simulink model "Sim1dot0"  (R2023b)
settings: Solver=VariableStepAuto  StartTime=0.0  StopTime=10.0  RelTol=1e-3
values from neighbouring files (symbols this model uses):
  dt = 0.02    [para_sim1dot0.mat]    (also in para_sim1dot1.mat; para_sim1dot2.mat; para_sim1dot3.mat; para_sim1dot4.mat)
  k_comp_1 = 1    [para_sim1dot0.mat]    (also in para_sim1dot1.mat; para_sim1dot2.mat; para_sim1dot3.mat; para_sim1dot4.mat)
  k_comp_2 = 1    [para_sim1dot0.mat]    (also in para_sim1dot1.mat; para_sim1dot2.mat; para_sim1dot3.mat; para_sim1dot4.mat)
  mass = 1    [para_sim1dot0.mat]    (also in para_sim1dot1.mat; para_sim1dot2.mat = 0.6; para_sim1dot3.mat = 0.8; para_sim1dot4.mat = 0.8)
  max_fin_angle_deg = 30    [para_sim1dot0.mat]    (also in para_sim1dot1.mat; para_sim1dot2.mat; para_sim1dot3.mat; para_sim1dot4.mat)
  v_min_controllable = 20    [para_sim1dot0.mat]    (also in para_sim1dot1.mat; para_sim1dot2.mat; para_sim1dot3.mat; para_sim1dot4.mat)
undefined symbols (not defined in the file or in its folder): DiscIntNeverNeededParam, state
libraries: robotcorelib x4, simulink x3, slpidlib x3, shared6dof x2, simulink_extras x2, aerolibutil x1, dspstat3 x1
settings Model: Creator=Zian Liu  LastModifiedBy=Zian Liu

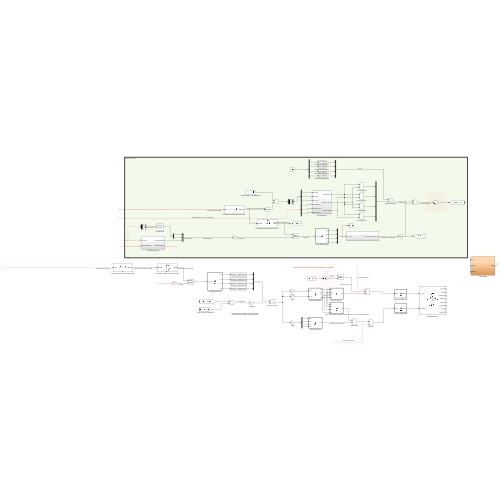
[thumbnail: Simulink's stored preview of the top-level diagram]
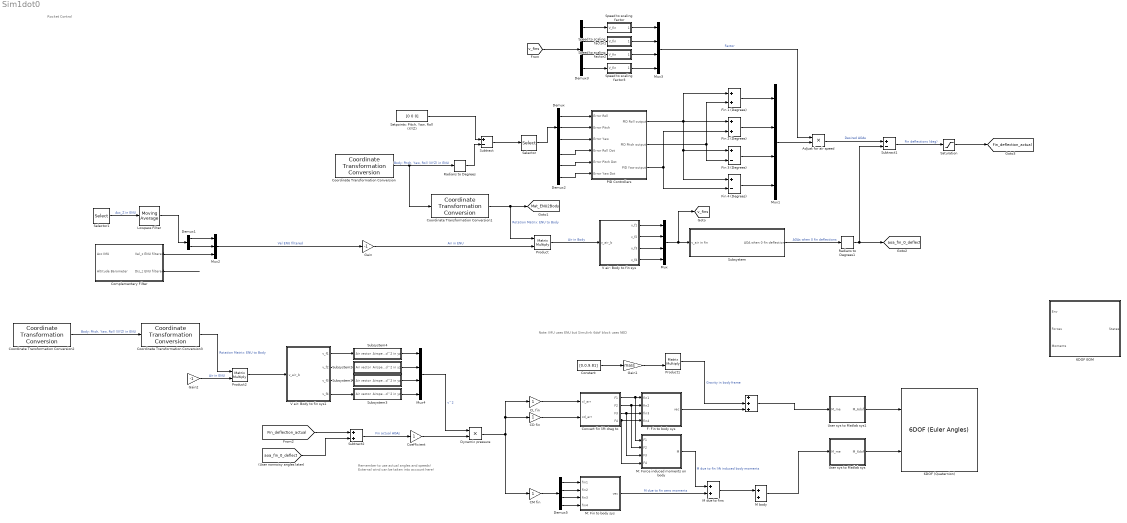
== system Sim1dot0 ==
  note: Note: IMU uses ENU but Simulink 6dof block uses NED
  note: Remember to use actual angles and speeds!
      | External wind can be taken into account here!
  note: Rocket Control
  " " : Sum  Inputs=+++
  6DOF (Quaternion) : shared6dof/6DOF (Euler Angles)  units=Metric (MKS)  mtype=Fixed  rep=Quaternion  xme_0=[0 0 0]  Vm_0=[0 0 0]  eul_0=[0 0 0]  pm_0=[0 0 0]  mass_0=1.0  mass_e=0.5  mass_f=2.0  inertia=eye(3)  inertia_e=eye(3)  inertia_f=2*eye(3)  k_quat=1.0  vre_flag=on  abi_flag=off  aMode=0  xme_statename=''  Vm_statename=''  eul_statename=''  quat_statename=''  pm_statename=''  mass_statename=''
      settings: LibrarySourceBlock=aerolib6dof2/6DOF (Quaternion)
  6DOF EOM : Subsystem  VariantControl=eom3DOF
  Adjust for air speed : Product
  CD fin : Gain
  CL fin : Gain
  CM fin : Gain
  Coefficient : Gain
  Complementary Filter : Subsystem
  Constant : Constant  Value=[0,0,9.81]
  "Convert fin lift drag to " : MATLAB Function  TreatAsAtomicUnit=on
  Coordinate Transformation Conversion : robotcorelib/Coordinate Transformation Conversion  InputRepresentation=Quaternion  InputEulerSequence=ZYX  ShowTrVecInputPort=on  OutputRepresentation=Euler Angles  OutputEulerSequence=XYZ  ShowTrVecOutputPort=on  SimulateUsing=Interpreted execution
      settings: LibrarySourceBlock=uavutilslib/Coordinate Transformation Conversion
  Coordinate Transformation Conversion1 : robotcorelib/Coordinate Transformation Conversion  InputRepresentation=Euler Angles  InputEulerSequence=XYZ  ShowTrVecInputPort=on  OutputRepresentation=Rotation Matrix  OutputEulerSequence=XYZ  ShowTrVecOutputPort=on  SimulateUsing=Interpreted execution
      settings: LibrarySourceBlock=uavutilslib/Coordinate Transformation Conversion
  Coordinate Transformation Conversion2 : robotcorelib/Coordinate Transformation Conversion  InputRepresentation=Quaternion  InputEulerSequence=ZYX  ShowTrVecInputPort=on  OutputRepresentation=Euler Angles  OutputEulerSequence=XYZ  ShowTrVecOutputPort=on  SimulateUsing=Interpreted execution
      settings: LibrarySourceBlock=uavutilslib/Coordinate Transformation Conversion
  Coordinate Transformation Conversion3 : robotcorelib/Coordinate Transformation Conversion  InputRepresentation=Euler Angles  InputEulerSequence=XYZ  ShowTrVecInputPort=on  OutputRepresentation=Rotation Matrix  OutputEulerSequence=XYZ  ShowTrVecOutputPort=on  SimulateUsing=Interpreted execution
      settings: LibrarySourceBlock=uavutilslib/Coordinate Transformation Conversion
  Demux : Demux  Outputs=3
  Demux1 : Demux  Outputs=2
  Demux2 : Demux  Outputs=3
  Demux3 : Demux
  Demux5 : Demux
  Dynamic pressure : Product
  F: Fin to body sys : MATLAB Function  TreatAsAtomicUnit=on
  Fin 1 (Degrees) : Sum
  Fin 2 (Degrees) : Sum
  Fin 3 (Degrees) : Sum  Inputs=+-
  Fin 4 (Degrees) : Sum  Inputs=+-
  Gain : Gain  Gain=-1
  Gain1 : Gain  Gain=mass
  Gain2 : Gain  Gain=-1
  Lowpass Filter : dspstat3/Moving Average  Method=Exponential weighting  ForgettingFactorPort=off  SpecifyWindowLength=on  WindowLength=4  OverlapLength=3  AllowArbitraryInputLength=off  ForgettingFactor=0.95  SimulateUsing=Code generation
  M body : Sum
  M due to fins : Sum
  M: Fin to body sys : MATLAB Function  TreatAsAtomicUnit=on
  M: Force induced moments on body : MATLAB Function  TreatAsAtomicUnit=on
  Mux{,1,3..4} (4 alike) : Mux
  Mux2 : Mux  Inputs=3
  PID Controllers : Subsystem
  Product : Product  Multiplication=Matrix(*)
  Product1 : Product  Multiplication=Matrix(*)
  Product2 : Product  Multiplication=Matrix(*)
  Radians to Degrees : simulink_extras/Transformations/Radians to Degrees
  Radians to Degrees1 : simulink_extras/Transformations/Radians to Degrees
  Saturation : Saturate  UpperLimit=max_fin_angle_deg  LowerLimit=-max_fin_angle_deg
  Selector : Selector  InputPortWidth=3  IndexOptions=Index vector (dialog)  Indices=[3 1 2]  OutputSizes=1
  Selector1 : Selector  InputPortWidth=3  IndexOptions=Index vector (dialog)  Indices=[1 2]  OutputSizes=1
  "Setpoints: Pitch, Yaw, Roll (XYZ)" : Constant  Value=[0 0 0]
  Speed to scaling factor : Subsystem
  Speed to scaling factor1 : Subsystem
  Speed to scaling factor2 : Subsystem
  Speed to scaling factor3 : Subsystem
  Subsystem : Subsystem
  Subsystem1 : Subsystem
  Subsystem2 : Subsystem
  Subsystem3 : Subsystem
  Subsystem4 : Subsystem
  Subtract : Sum  Inputs=+-
  Subtract1 : Sum  Inputs=+-
  Subtract2 : Sum
  User sys to Matlab sys : MATLAB Function  TreatAsAtomicUnit=on
  User sys to Matlab sys1 : MATLAB Function  TreatAsAtomicUnit=on
  V air: Body to fin sys : MATLAB Function  TreatAsAtomicUnit=on
  V air: Body to fin sys1 : MATLAB Function  TreatAsAtomicUnit=on
  tag scope: Fin_deflection_actual=global, Mat_ENU2Body=global, aoa_fin_0_deflect=global, v_fins=global
  wires:
  ? -> Coordinate Transformation Conversion/1  "Rocket attitude in quaternion"
  Coordinate Transformation Conversion/1 -> Coordinate Transformation Conversion1/1, Radians to Degrees/1  "Body: Pitch, Yaw, Roll (XYZ) in ENU"
  "Setpoints: Pitch, Yaw, Roll (XYZ)"/1 -> Subtract/1
  Subtract/1 -> Selector/1
  Selector/1 -> Demux/1
  Fin 1 (Degrees)/1 -> Mux1/1
  Fin 2 (Degrees)/1 -> Mux1/2
  Fin 3 (Degrees)/1 -> Mux1/3
  Fin 4 (Degrees)/1 -> Mux1/4
  Radians to Degrees/1 -> Subtract/2
  Gain/1 -> Product/2  "Air in ENU"
  Coordinate Transformation Conversion1/1 -> [Mat_ENU2Body], Product/1  "Rotation Matrix: ENU to Body"
  Product/1 -> V air: Body to fin sys/1(v_air_b)  "Air in Body"
  V air: Body to fin sys/4(v_f4) -> Mux/4
  V air: Body to fin sys/3(v_f3) -> Mux/3
  V air: Body to fin sys/2(v_f2) -> Mux/2
  V air: Body to fin sys/1(v_f1) -> Mux/1
  Mux/1 -> [v_fins], Subsystem/1(v_air in fin)
  Mux3/1 -> Adjust for air speed/1  "Factor"
  Mux1/1 -> Adjust for air speed/2
  Adjust for air speed/1 -> Subtract1/1  "Desired AOAs"
  Subsystem/1(AOA when 0 fin deflection) -> Radians to Degrees1/1  "AOAs when 0 fin deflections"
  Subtract1/1 -> Saturation/1  "Fin deflections (deg)"
  Saturation/1 -> [Fin_deflection_actual]
  Complementary Filter/1(Vel_z ENU filtered) -> Mux2/3
  ? -> Demux2/1  "Rocket angular rates in rad/s, body frame"
  Complementary Filter/2(Dis_z ENU filtered) -> ?
  ? -> Complementary Filter/2(Altitude Barometer)
  ? -> Selector1/1, Complementary Filter/1(Acc IMU)
  Selector1/1 -> Lowpass Filter/1  "Acc_Z in ENU"
  Lowpass Filter/1 -> Demux1/1
  Demux1/1 -> Mux2/1
  Demux1/2 -> Mux2/2
  Mux2/1 -> Gain/1  "Vel ENU filtered"
  PID Controllers/3(PID Yaw output) -> Fin 2 (Degrees)/2, Fin 4 (Degrees)/2
  PID Controllers/1(PID Roll output) -> Fin 4 (Degrees)/1, Fin 3 (Degrees)/1, Fin 2 (Degrees)/1, Fin 1 (Degrees)/1
  PID Controllers/2(PID Pitch output) -> Fin 1 (Degrees)/2, Fin 3 (Degrees)/2
  Demux/1 -> PID Controllers/1(Error Roll)
  Demux/2 -> PID Controllers/2(Error Pitch)
  Demux/3 -> PID Controllers/3(Error Yaw)
  Demux2/1 -> PID Controllers/4(Error Roll Dot)
  Demux2/2 -> PID Controllers/5(Error Pitch Dot)
  Demux2/3 -> PID Controllers/6(Error Yaw Dot)
  [aoa_fin_0_deflect] -> Subtract2/2
  Subtract2/1 -> Coefficient/1  "Fin actual AOAs"
  Radians to Degrees1/1 -> Subtract1/2, [aoa_fin_0_deflect]
  Coefficient/1 -> Dynamic pressure/2
  [v_fins] -> Demux3/1
  Demux3/1 -> Speed to scaling factor/1(V_fin)
  Demux3/4 -> Speed to scaling factor3/1(V_fin)
  Demux3/3 -> Speed to scaling factor2/1(V_fin)
  Demux3/2 -> Speed to scaling factor1/1(V_fin)
  Speed to scaling factor3/1(Factor) -> Mux3/4
  Speed to scaling factor2/1(Factor) -> Mux3/3
  Speed to scaling factor1/1(Factor) -> Mux3/2
  Speed to scaling factor/1(Factor) -> Mux3/1
  V air: Body to fin sys1/4(v_f4) -> Subsystem3/1(Air vector)
  V air: Body to fin sys1/3(v_f3) -> Subsystem1/1(Air vector)
  V air: Body to fin sys1/2(v_f2) -> Subsystem2/1(Air vector)
  V air: Body to fin sys1/1(v_f1) -> Subsystem4/1(Air vector)
  Subsystem4/1(Airspeed^2 in yz) -> Mux4/1
  Subsystem2/1(Airspeed^2 in yz) -> Mux4/2
  Subsystem1/1(Airspeed^2 in yz) -> Mux4/3
  Subsystem3/1(Airspeed^2 in yz) -> Mux4/4
  Mux4/1 -> Dynamic pressure/1  "v^2"
  Dynamic pressure/1 -> CL fin/1, CD fin/1, CM fin/1
  CL fin/1 -> "Convert fin lift drag to "/1(cl_arr)
  CM fin/1 -> Demux5/1
  F: Fin to body sys/1(vec) -> " "/3
  [Fin_deflection_actual] -> Subtract2/1
  "Convert fin lift drag to "/2(F2) -> M: Force induced moments on body/2(F2), F: Fin to body sys/2(fin2)
  "Convert fin lift drag to "/3(F3) -> M: Force induced moments on body/3(F3), F: Fin to body sys/3(fin3)
  "Convert fin lift drag to "/4(F4) -> M: Force induced moments on body/4(F4), F: Fin to body sys/4(fin4)
  CD fin/1 -> "Convert fin lift drag to "/2(cd_arr)
  Demux5/1 -> M: Fin to body sys/1(fin1)
  Demux5/2 -> M: Fin to body sys/2(fin2)
  Demux5/4 -> M: Fin to body sys/4(fin4)
  Demux5/3 -> M: Fin to body sys/3(fin3)
  "Convert fin lift drag to "/1(F1) -> M: Force induced moments on body/1(F1), F: Fin to body sys/1(fin1)
  M: Force induced moments on body/1(M) -> M due to fins/1  "M due to fin lift induced body moments"
  M: Fin to body sys/1(vec) -> M due to fins/2  "M due to fin aero moments"
  Constant/1 -> Gain1/1
  Gain1/1 -> Product1/2
  ? -> Product1/1  "DCM"
  Product1/1 -> " "/2  "Gravity in body frame"
  M due to fins/1 -> M body/1
  M body/1 -> User sys to Matlab sys/1(M_me)
  ? -> " "/1  "F due to rocket body"
  ? -> M body/2  "M due to rocket body"
  User sys to Matlab sys/1(M_6dof) -> 6DOF (Quaternion)/2
  User sys to Matlab sys1/1(M_6dof) -> 6DOF (Quaternion)/1
  " "/1 -> User sys to Matlab sys1/1(M_me)
  Product2/1 -> V air: Body to fin sys1/1(v_air_b)
  ? -> Coordinate Transformation Conversion2/1  "Rocket attitude in quaternion"
  Coordinate Transformation Conversion2/1 -> Coordinate Transformation Conversion3/1  "Body: Pitch, Yaw, Roll (XYZ) in ENU"
  Coordinate Transformation Conversion3/1 -> Product2/1  "Rotation Matrix: ENU to Body"
  ? -> Gain2/1
  Gain2/1 -> Product2/2  "Air in ENU"

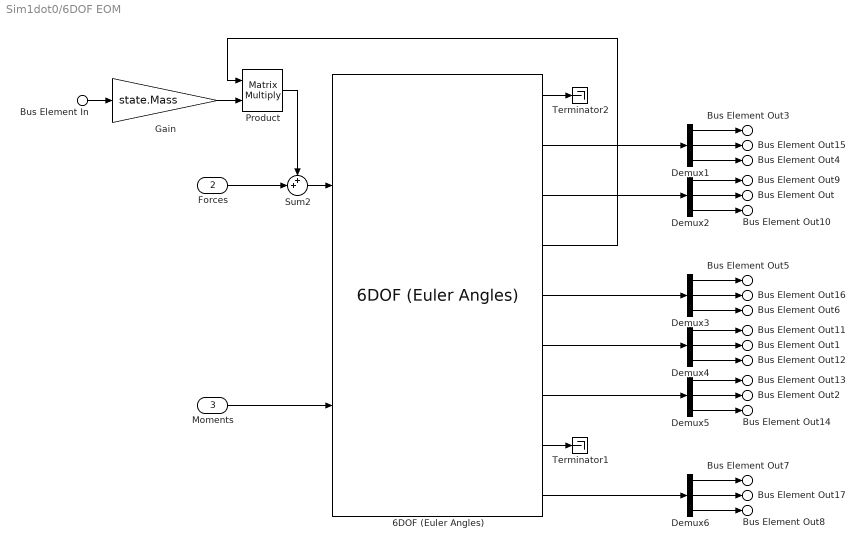
== system Sim1dot0/6DOF EOM ==
  Bus Element In : Inport  PortName=Env  Element=g
  Forces : Inport  Port=2
  Moments : Inport  Port=3
  6DOF (Euler Angles) : shared6dof/6DOF (Euler Angles)  units=Metric (MKS)  mtype=Fixed  rep=Quaternion  xme_0=[state.XN, state.XE, state.XD]  Vm_0=[state.U, state.V, state.W]  eul_0=[state.Phi, state.Theta, state.Psi]  pm_0=[state.P, state.Q, state.R]  mass_0=state.Mass  mass_e=0.5  mass_f=2.0  inertia=state.Inertia.Variables  inertia_e=eye(3)  inertia_f=2*eye(3)  k_quat=1.0  vre_flag=on  abi_flag=on  aMode=0  xme_statename={'Xe', 'Ye', 'Ze'}  Vm_statename={'U', 'V', 'W'}  eul_statename={'phi', 'theta', 'psi'}  quat_statename={'qr', 'qi', 'qj','qk'}  pm_statename={'p', 'q', 'r'}  mass_statename=''
  Demux{1..6} (6 alike) : Demux  Outputs=3
  Gain : Gain  Gain=state.Mass
  Product : Product  Multiplication=Matrix(*)
  Sum2 : Sum  Inputs=++|  InputSameDT=on  SaturateOnIntegerOverflow=on  OutDataTypeStr=Inherit: Same as first input
  Terminator1 : Terminator
  Terminator2 : Terminator
  Bus Element Out3 : Outport  VectorParamsAs1DForOutWhenUnconnected=off  PortName=States  Element=Xe
  Bus Element Out4 : Outport  VectorParamsAs1DForOutWhenUnconnected=off  PortName=States  Element=Ze
  Bus Element Out : Outport  VectorParamsAs1DForOutWhenUnconnected=off  PortName=States  Element=theta
  Bus Element Out5 : Outport  VectorParamsAs1DForOutWhenUnconnected=off  PortName=States  Element=u
  Bus Element Out6 : Outport  VectorParamsAs1DForOutWhenUnconnected=off  PortName=States  Element=w
  Bus Element Out1 : Outport  VectorParamsAs1DForOutWhenUnconnected=off  PortName=States  Element=q
  Bus Element Out2 : Outport  VectorParamsAs1DForOutWhenUnconnected=off  PortName=States  Element=q_dot
  Bus Element Out7 : Outport  VectorParamsAs1DForOutWhenUnconnected=off  PortName=States  Element=Axe
  Bus Element Out8 : Outport  VectorParamsAs1DForOutWhenUnconnected=off  PortName=States  Element=Aze
  Bus Element Out15 : Outport  VectorParamsAs1DForOutWhenUnconnected=off  PortName=States  Element=Ye
  Bus Element Out9 : Outport  VectorParamsAs1DForOutWhenUnconnected=off  PortName=States  Element=phi
  Bus Element Out10 : Outport  VectorParamsAs1DForOutWhenUnconnected=off  PortName=States  Element=psi
  Bus Element Out16 : Outport  VectorParamsAs1DForOutWhenUnconnected=off  PortName=States  Element=v
  Bus Element Out11 : Outport  VectorParamsAs1DForOutWhenUnconnected=off  PortName=States  Element=p
  Bus Element Out12 : Outport  VectorParamsAs1DForOutWhenUnconnected=off  PortName=States  Element=r
  Bus Element Out13 : Outport  VectorParamsAs1DForOutWhenUnconnected=off  PortName=States  Element=p_dot
  Bus Element Out14 : Outport  VectorParamsAs1DForOutWhenUnconnected=off  PortName=States  Element=r_dot
  Bus Element Out17 : Outport  VectorParamsAs1DForOutWhenUnconnected=off  PortName=States  Element=Aye
  wires:
  6DOF (Euler Angles)/2 -> Demux1/1
  6DOF (Euler Angles)/4 -> Product/1
  6DOF (Euler Angles)/1 -> Terminator2/1
  Bus Element In/1 -> Gain/1
  Demux6/2 -> Bus Element Out17/1
  Demux6/3 -> Bus Element Out8/1
  Demux6/1 -> Bus Element Out7/1
  6DOF (Euler Angles)/9 -> Demux6/1
  6DOF (Euler Angles)/7 -> Demux5/1
  Demux5/3 -> Bus Element Out14/1
  Demux5/2 -> Bus Element Out2/1
  Demux5/1 -> Bus Element Out13/1
  6DOF (Euler Angles)/6 -> Demux4/1
  Demux4/3 -> Bus Element Out12/1
  Demux4/2 -> Bus Element Out1/1
  Demux4/1 -> Bus Element Out11/1
  Demux3/3 -> Bus Element Out6/1
  Demux3/2 -> Bus Element Out16/1
  Demux3/1 -> Bus Element Out5/1
  6DOF (Euler Angles)/5 -> Demux3/1
  Demux2/3 -> Bus Element Out10/1
  Demux2/2 -> Bus Element Out/1
  Demux2/1 -> Bus Element Out9/1
  Demux1/1 -> Bus Element Out3/1
  Demux1/3 -> Bus Element Out4/1
  Demux1/2 -> Bus Element Out15/1
  Gain/1 -> Product/2
  6DOF (Euler Angles)/3 -> Demux2/1
  Moments/1 -> 6DOF (Euler Angles)/2
  Forces/1 -> Sum2/2
  Sum2/1 -> 6DOF (Euler Angles)/1
  Product/1 -> Sum2/1
  6DOF (Euler Angles)/8 -> Terminator1/1

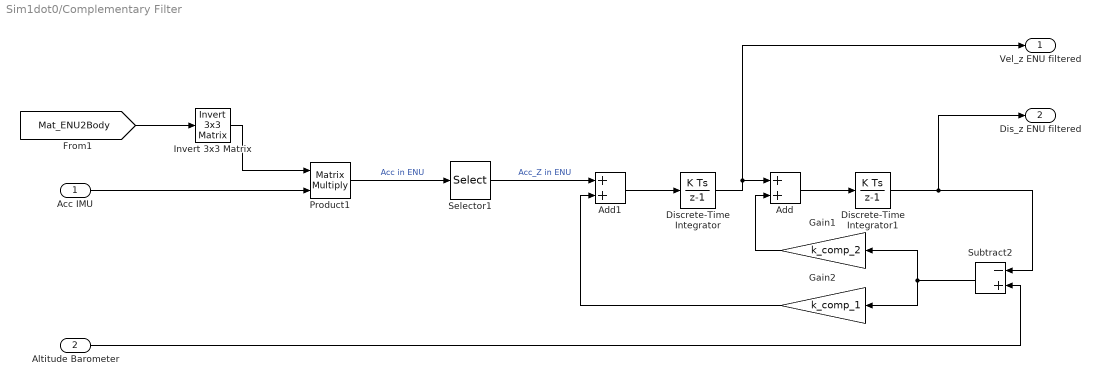
== system Sim1dot0/Complementary Filter ==
  Acc IMU : Inport
  Altitude Barometer : Inport  Port=2
  Add : Sum
  Add1 : Sum
  Discrete-Time Integrator : DiscreteIntegrator  SampleTime=-1  ICPrevOutput=DiscIntNeverNeededParam  ICPrevScaledInput=DiscIntNeverNeededParam
  Discrete-Time Integrator1 : DiscreteIntegrator  SampleTime=-1  ICPrevOutput=DiscIntNeverNeededParam  ICPrevScaledInput=DiscIntNeverNeededParam
  Gain1 : Gain  Gain=k_comp_2
  Gain2 : Gain  Gain=k_comp_1
  Invert 3x3 Matrix : aerolibutil/Invert  3x3 Matrix
  Product1 : Product  Multiplication=Matrix(*)
  Selector1 : Selector  InputPortWidth=3  IndexOptions=Index vector (dialog)  Indices=3  OutputSizes=1
  Subtract2 : Sum  Inputs=-+
  Vel_z ENU filtered : Outport
  Dis_z ENU filtered : Outport  Port=2
  wires:
  [Mat_ENU2Body] -> Invert 3x3 Matrix/1
  Product1/1 -> Selector1/1  "Acc in ENU"
  Subtract2/1 -> Gain1/1, Gain2/1
  Discrete-Time Integrator1/1 -> Subtract2/1, Dis_z ENU filtered/1
  Gain1/1 -> Add/2
  Add/1 -> Discrete-Time Integrator1/1
  Discrete-Time Integrator/1 -> Vel_z ENU filtered/1, Add/1
  Selector1/1 -> Add1/1  "Acc_Z in ENU"
  Add1/1 -> Discrete-Time Integrator/1
  Gain2/1 -> Add1/2
  Acc IMU/1 -> Product1/2
  Invert 3x3 Matrix/1 -> Product1/1
  Altitude Barometer/1 -> Subtract2/2

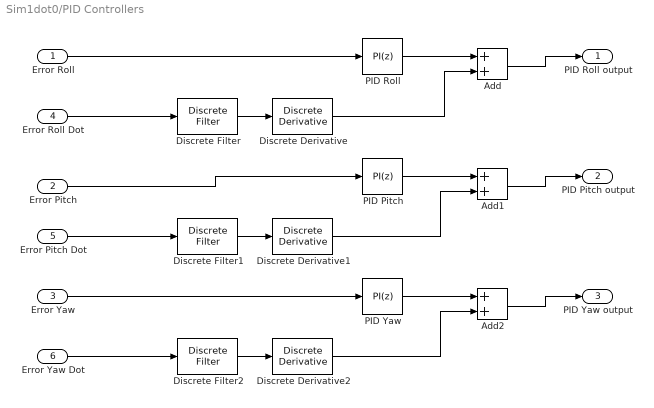
== system Sim1dot0/PID Controllers ==
  Error Roll : Inport
  Error Pitch : Inport  Port=2
  Error Yaw : Inport  Port=3
  Error Roll Dot : Inport  Port=4
  Error Pitch Dot : Inport  Port=5
  Error Yaw Dot : Inport  Port=6
  Add : Sum
  Add1 : Sum
  Add2 : Sum
  Discrete Derivative : simulink/Discrete/Discrete Derivative  gainval=1.0  ICPrevScaledInput=0.0  OutMin=[]  OutMax=[]  OutDataType=fixdt(1, 16)  OutScaling=2^-10  DoSatur=off
  Discrete Derivative1 : simulink/Discrete/Discrete Derivative  gainval=1.0  ICPrevScaledInput=0.0  OutMin=[]  OutMax=[]  OutDataType=fixdt(1, 16)  OutScaling=2^-10  DoSatur=off
  Discrete Derivative2 : simulink/Discrete/Discrete Derivative  gainval=1.0  ICPrevScaledInput=0.0  OutMin=[]  OutMax=[]  OutDataType=fixdt(1, 16)  OutScaling=2^-10  DoSatur=off
  Discrete Filter : DiscreteFilter
  Discrete Filter1 : DiscreteFilter
  Discrete Filter2 : DiscreteFilter
  PID Pitch : slpidlib/PID Controller  Controller=PI  Form=Parallel  TimeDomain=Discrete-time  UseExternalTs=off  SampleTime=dt  IntegratorMethod=Forward Euler  FilterMethod=Forward Euler  ControllerParametersSource=internal  P=1  I=1  UseKiTs=off  D=0  N=100  UseFilter=on  TunerSelectOption=Transfer Function Based (PID Tuner App)  InitialConditionSource=internal  InitialConditionForIntegrator=0  InitialConditionForFilter=0  DifferentiatorICPrevScaledInput=0  ExternalReset=none  TrackingMode=off  Kt=1  LimitOutput=off  SatLimitsSource=internal  UpperSaturationLimit=inf  LowerSaturationLimit=-inf  LinearizeAsGain=on  AntiWindupMode=none  Kb=1  LimitIntegrator=off  UpperIntegratorSaturationLimit=inf  LowerIntegratorSaturationLimit=-inf  POutMin=[]  POutMax=[]  IOutMin=[]  IOutMax=[]  DOutMin=[]  DOutMax=[]  NOutMin=[]  NOutMax=[]  SumOutMin=[]  SumOutMax=[]  SaturationOutMin=[]  SaturationOutMax=[]  PParamMin=[]  PParamMax=[]  IParamMin=[]  IParamMax=[]  DParamMin=[]  DParamMax=[]  NParamMin=[]  NParamMax=[]  KbParamMin=[]  KbParamMax=[]  KtParamMin=[]  KtParamMax=[]  KbOutMin=[]  KbOutMax=[]  KtOutMin=[]  KtOutMax=[]  IntegratorOutMin=[]  IntegratorOutMax=[]  FilterOutMin=[]  FilterOutMax=[]  SumI1OutMin=[]  SumI1OutMax=[]  SumI2OutMin=[]  SumI2OutMax=[]  SumI3OutMin=[]  SumI3OutMax=[]  SumI4OutMin=[]  SumI4OutMax=[]  SumDOutMin=[]  SumDOutMax=[]  DifferentiatorOutMin=[]  DifferentiatorOutMax=[]  FilterDiffOutCoefMin=[]  FilterDiffOutCoefMax=[]  ReciprocalOutMin=[]  ReciprocalOutMax=[]  SumDenOutMin=[]  SumDenOutMax=[]  SumNumOutMin=[]  SumNumOutMax=[]  DivideOutMin=[]  DivideOutMax=[]  UdiffTsProdOutMin=[]  UdiffTsProdOutMax=[]  NTsProdOutMin=[]  NTsProdOutMax=[]  UintegralTsProdOutMin=[]  UintegralTsProdOutMax=[]  UngainTsProdOutMin=[]  UngainTsProdOutMax=[]  ClampingZeroOutDataTypeStr=Inherit: Inherit via back propagation  ClampingZeroOutMin=[]  ClampingZeroOutMax=[]  FilterDenConstantOutDataTypeStr=Inherit: Inherit via back propagation  FilterDenConstantOutMin=[]  FilterDenConstantOutMax=[]  PCopyOutDataTypeStr=Inherit: Inherit via back propagation  PCopyOutMin=[]  PCopyOutMax=[]  NCopyOutDataTypeStr=Inherit: Inherit via back propagation  NCopyOutMin=[]  NCopyOutMax=[]  IntegratorContinuousStateAttributes=''  IntegratorStateMustResolveToSignalObject=off  IntegratorRTWStateStorageClass=Auto  FilterContinuousStateAttributes=''  FilterStateMustResolveToSignalObject=off  FilterRTWStateStorageClass=Auto  ParallelPVariant=InternalParameters  IdealPVariant=Disabled  IVariant=InternalParameters  DVariant=Disabled  IntegratorVariant=Discrete  SatVariant=Disabled  AWVariant=Passthrough  PCopyVariant=Disabled  TRVariant=Disabled  FdbkBlocksVariant=Forward  IdealPFdbkVariant=Disabled  SatFdbkVariant=Disabled  DerivativeFilterVariant=Disabled  NVariant=Disabled  NCopyVariant=Disabled_SignalSpec  FilterICVariant=Disabled  IntegratorICVariant=InternalICs  ExternalResetVariant=Disabled  TRSumVariant=Passthrough  SumFdbkVariant=Disabled  SumVariant=Sum_PI  TsampFilterVariant=InternalTs  TsampNgainVariant=Passthrough  TsampIntegralVariant=Disabled_SignalSpec  ExternalSaturationOutDataTypeStr=Inherit: Same as second input
  PID Roll : slpidlib/PID Controller  Controller=PI  Form=Parallel  TimeDomain=Discrete-time  UseExternalTs=off  SampleTime=dt  IntegratorMethod=Forward Euler  FilterMethod=Forward Euler  ControllerParametersSource=internal  P=1  I=1  UseKiTs=off  D=0  N=100  UseFilter=on  TunerSelectOption=Transfer Function Based (PID Tuner App)  InitialConditionSource=internal  InitialConditionForIntegrator=0  InitialConditionForFilter=0  DifferentiatorICPrevScaledInput=0  ExternalReset=none  TrackingMode=off  Kt=1  LimitOutput=off  SatLimitsSource=internal  UpperSaturationLimit=inf  LowerSaturationLimit=-inf  LinearizeAsGain=on  AntiWindupMode=none  Kb=1  LimitIntegrator=off  UpperIntegratorSaturationLimit=inf  LowerIntegratorSaturationLimit=-inf  POutMin=[]  POutMax=[]  IOutMin=[]  IOutMax=[]  DOutMin=[]  DOutMax=[]  NOutMin=[]  NOutMax=[]  SumOutMin=[]  SumOutMax=[]  SaturationOutMin=[]  SaturationOutMax=[]  PParamMin=[]  PParamMax=[]  IParamMin=[]  IParamMax=[]  DParamMin=[]  DParamMax=[]  NParamMin=[]  NParamMax=[]  KbParamMin=[]  KbParamMax=[]  KtParamMin=[]  KtParamMax=[]  KbOutMin=[]  KbOutMax=[]  KtOutMin=[]  KtOutMax=[]  IntegratorOutMin=[]  IntegratorOutMax=[]  FilterOutMin=[]  FilterOutMax=[]  SumI1OutMin=[]  SumI1OutMax=[]  SumI2OutMin=[]  SumI2OutMax=[]  SumI3OutMin=[]  SumI3OutMax=[]  SumI4OutMin=[]  SumI4OutMax=[]  SumDOutMin=[]  SumDOutMax=[]  DifferentiatorOutMin=[]  DifferentiatorOutMax=[]  FilterDiffOutCoefMin=[]  FilterDiffOutCoefMax=[]  ReciprocalOutMin=[]  ReciprocalOutMax=[]  SumDenOutMin=[]  SumDenOutMax=[]  SumNumOutMin=[]  SumNumOutMax=[]  DivideOutMin=[]  DivideOutMax=[]  UdiffTsProdOutMin=[]  UdiffTsProdOutMax=[]  NTsProdOutMin=[]  NTsProdOutMax=[]  UintegralTsProdOutMin=[]  UintegralTsProdOutMax=[]  UngainTsProdOutMin=[]  UngainTsProdOutMax=[]  ClampingZeroOutDataTypeStr=Inherit: Inherit via back propagation  ClampingZeroOutMin=[]  ClampingZeroOutMax=[]  FilterDenConstantOutDataTypeStr=Inherit: Inherit via back propagation  FilterDenConstantOutMin=[]  FilterDenConstantOutMax=[]  PCopyOutDataTypeStr=Inherit: Inherit via back propagation  PCopyOutMin=[]  PCopyOutMax=[]  NCopyOutDataTypeStr=Inherit: Inherit via back propagation  NCopyOutMin=[]  NCopyOutMax=[]  IntegratorContinuousStateAttributes=''  IntegratorStateMustResolveToSignalObject=off  IntegratorRTWStateStorageClass=Auto  FilterContinuousStateAttributes=''  FilterStateMustResolveToSignalObject=off  FilterRTWStateStorageClass=Auto  ParallelPVariant=InternalParameters  IdealPVariant=Disabled  IVariant=InternalParameters  DVariant=Disabled  IntegratorVariant=Discrete  SatVariant=Disabled  AWVariant=Passthrough  PCopyVariant=Disabled  TRVariant=Disabled  FdbkBlocksVariant=Forward  IdealPFdbkVariant=Disabled  SatFdbkVariant=Disabled  DerivativeFilterVariant=Disabled  NVariant=Disabled  NCopyVariant=Disabled_SignalSpec  FilterICVariant=Disabled  IntegratorICVariant=InternalICs  ExternalResetVariant=Disabled  TRSumVariant=Passthrough  SumFdbkVariant=Disabled  SumVariant=Sum_PI  TsampFilterVariant=InternalTs  TsampNgainVariant=Passthrough  TsampIntegralVariant=Disabled_SignalSpec  ExternalSaturationOutDataTypeStr=Inherit: Same as second input
  PID Yaw : slpidlib/PID Controller  Controller=PI  Form=Parallel  TimeDomain=Discrete-time  UseExternalTs=off  SampleTime=dt  IntegratorMethod=Forward Euler  FilterMethod=Forward Euler  ControllerParametersSource=internal  P=1  I=1  UseKiTs=off  D=0  N=100  UseFilter=on  TunerSelectOption=Transfer Function Based (PID Tuner App)  InitialConditionSource=internal  InitialConditionForIntegrator=0  InitialConditionForFilter=0  DifferentiatorICPrevScaledInput=0  ExternalReset=none  TrackingMode=off  Kt=1  LimitOutput=off  SatLimitsSource=internal  UpperSaturationLimit=inf  LowerSaturationLimit=-inf  LinearizeAsGain=on  AntiWindupMode=none  Kb=1  LimitIntegrator=off  UpperIntegratorSaturationLimit=inf  LowerIntegratorSaturationLimit=-inf  POutMin=[]  POutMax=[]  IOutMin=[]  IOutMax=[]  DOutMin=[]  DOutMax=[]  NOutMin=[]  NOutMax=[]  SumOutMin=[]  SumOutMax=[]  SaturationOutMin=[]  SaturationOutMax=[]  PParamMin=[]  PParamMax=[]  IParamMin=[]  IParamMax=[]  DParamMin=[]  DParamMax=[]  NParamMin=[]  NParamMax=[]  KbParamMin=[]  KbParamMax=[]  KtParamMin=[]  KtParamMax=[]  KbOutMin=[]  KbOutMax=[]  KtOutMin=[]  KtOutMax=[]  IntegratorOutMin=[]  IntegratorOutMax=[]  FilterOutMin=[]  FilterOutMax=[]  SumI1OutMin=[]  SumI1OutMax=[]  SumI2OutMin=[]  SumI2OutMax=[]  SumI3OutMin=[]  SumI3OutMax=[]  SumI4OutMin=[]  SumI4OutMax=[]  SumDOutMin=[]  SumDOutMax=[]  DifferentiatorOutMin=[]  DifferentiatorOutMax=[]  FilterDiffOutCoefMin=[]  FilterDiffOutCoefMax=[]  ReciprocalOutMin=[]  ReciprocalOutMax=[]  SumDenOutMin=[]  SumDenOutMax=[]  SumNumOutMin=[]  SumNumOutMax=[]  DivideOutMin=[]  DivideOutMax=[]  UdiffTsProdOutMin=[]  UdiffTsProdOutMax=[]  NTsProdOutMin=[]  NTsProdOutMax=[]  UintegralTsProdOutMin=[]  UintegralTsProdOutMax=[]  UngainTsProdOutMin=[]  UngainTsProdOutMax=[]  ClampingZeroOutDataTypeStr=Inherit: Inherit via back propagation  ClampingZeroOutMin=[]  ClampingZeroOutMax=[]  FilterDenConstantOutDataTypeStr=Inherit: Inherit via back propagation  FilterDenConstantOutMin=[]  FilterDenConstantOutMax=[]  PCopyOutDataTypeStr=Inherit: Inherit via back propagation  PCopyOutMin=[]  PCopyOutMax=[]  NCopyOutDataTypeStr=Inherit: Inherit via back propagation  NCopyOutMin=[]  NCopyOutMax=[]  IntegratorContinuousStateAttributes=''  IntegratorStateMustResolveToSignalObject=off  IntegratorRTWStateStorageClass=Auto  FilterContinuousStateAttributes=''  FilterStateMustResolveToSignalObject=off  FilterRTWStateStorageClass=Auto  ParallelPVariant=InternalParameters  IdealPVariant=Disabled  IVariant=InternalParameters  DVariant=Disabled  IntegratorVariant=Discrete  SatVariant=Disabled  AWVariant=Passthrough  PCopyVariant=Disabled  TRVariant=Disabled  FdbkBlocksVariant=Forward  IdealPFdbkVariant=Disabled  SatFdbkVariant=Disabled  DerivativeFilterVariant=Disabled  NVariant=Disabled  NCopyVariant=Disabled_SignalSpec  FilterICVariant=Disabled  IntegratorICVariant=InternalICs  ExternalResetVariant=Disabled  TRSumVariant=Passthrough  SumFdbkVariant=Disabled  SumVariant=Sum_PI  TsampFilterVariant=InternalTs  TsampNgainVariant=Passthrough  TsampIntegralVariant=Disabled_SignalSpec  ExternalSaturationOutDataTypeStr=Inherit: Same as second input
  PID Roll output : Outport
  PID Pitch output : Outport  Port=2
  PID Yaw output : Outport  Port=3
  wires:
  PID Pitch/1 -> Add1/1
  PID Roll/1 -> Add/1
  Error Pitch/1 -> PID Pitch/1
  PID Yaw/1 -> Add2/1
  Error Yaw/1 -> PID Yaw/1
  Error Roll/1 -> PID Roll/1
  Discrete Filter/1 -> Discrete Derivative/1
  Discrete Filter1/1 -> Discrete Derivative1/1
  Discrete Derivative1/1 -> Add1/2
  Discrete Derivative/1 -> Add/2
  Discrete Derivative2/1 -> Add2/2
  Discrete Filter2/1 -> Discrete Derivative2/1
  Add/1 -> PID Roll output/1
  Add1/1 -> PID Pitch output/1
  Add2/1 -> PID Yaw output/1
  Error Roll Dot/1 -> Discrete Filter/1
  Error Pitch Dot/1 -> Discrete Filter1/1
  Error Yaw Dot/1 -> Discrete Filter2/1

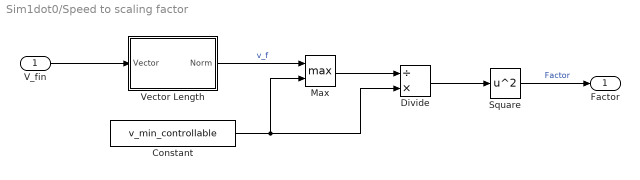
== system Sim1dot0/Speed to scaling factor ==
  V_fin : Inport
  Constant : Constant  Value=v_min_controllable
  Divide : Product  Inputs=/*
  Max : MinMax  Function=max  Inputs=2
  Square : Math  Operator=square
  Vector Length : Subsystem
  Factor : Outport
  wires:
  V_fin/1 -> Vector Length/1(Vector)
  Vector Length/1(Norm) -> Max/1  "v_f"
  Max/1 -> Divide/1
  Constant/1 -> Max/2, Divide/2
  Divide/1 -> Square/1
  Square/1 -> Factor/1  "Factor"

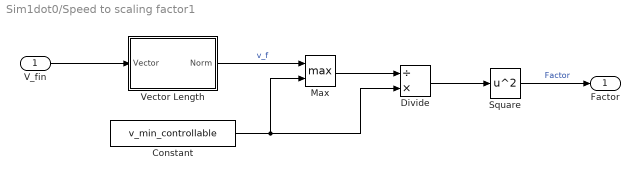
== system Sim1dot0/Speed to scaling factor1 ==
  V_fin : Inport
  Constant : Constant  Value=v_min_controllable
  Divide : Product  Inputs=/*
  Max : MinMax  Function=max  Inputs=2
  Square : Math  Operator=square
  Vector Length : Subsystem
  Factor : Outport
  wires:
  V_fin/1 -> Vector Length/1(Vector)
  Vector Length/1(Norm) -> Max/1  "v_f"
  Max/1 -> Divide/1
  Constant/1 -> Max/2, Divide/2
  Divide/1 -> Square/1
  Square/1 -> Factor/1  "Factor"

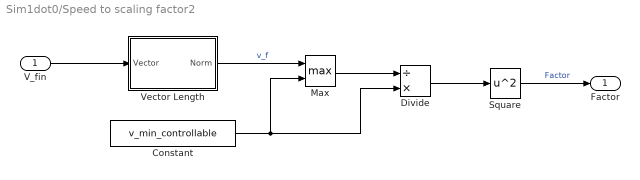
== system Sim1dot0/Speed to scaling factor2 ==
  V_fin : Inport
  Constant : Constant  Value=v_min_controllable
  Divide : Product  Inputs=/*
  Max : MinMax  Function=max  Inputs=2
  Square : Math  Operator=square
  Vector Length : Subsystem
  Factor : Outport
  wires:
  V_fin/1 -> Vector Length/1(Vector)
  Vector Length/1(Norm) -> Max/1  "v_f"
  Max/1 -> Divide/1
  Constant/1 -> Max/2, Divide/2
  Divide/1 -> Square/1
  Square/1 -> Factor/1  "Factor"

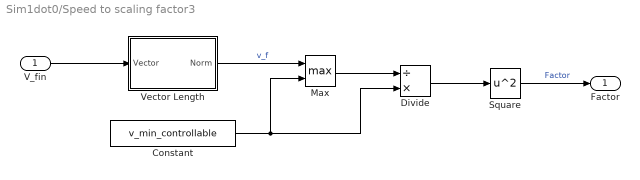
== system Sim1dot0/Speed to scaling factor3 ==
  V_fin : Inport
  Constant : Constant  Value=v_min_controllable
  Divide : Product  Inputs=/*
  Max : MinMax  Function=max  Inputs=2
  Square : Math  Operator=square
  Vector Length : Subsystem
  Factor : Outport
  wires:
  V_fin/1 -> Vector Length/1(Vector)
  Vector Length/1(Norm) -> Max/1  "v_f"
  Max/1 -> Divide/1
  Constant/1 -> Max/2, Divide/2
  Divide/1 -> Square/1
  Square/1 -> Factor/1  "Factor"

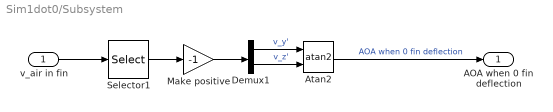
== system Sim1dot0/Subsystem ==
  v_air in fin : Inport
  Atan2 : Trigonometry  Operator=atan2
  Demux1 : Demux  Outputs=2
  Make positive : Gain  Gain=-1
  Selector1 : Selector  InputPortWidth=3  IndexOptions=Index vector (dialog)  Indices=[2 3]  OutputSizes=1
  AOA when 0 fin deflection : Outport
  wires:
  Demux1/2 -> Atan2/2  "v_z'"
  Demux1/1 -> Atan2/1  "v_y'"
  Selector1/1 -> Make positive/1
  Atan2/1 -> AOA when 0 fin deflection/1  "AOA when 0 fin deflection"
  Make positive/1 -> Demux1/1
  v_air in fin/1 -> Selector1/1

== system Sim1dot0/Subsystem1 ==
  Air vector : Inport
  Selector2 : Selector  InputPortWidth=3  IndexOptions=Index vector (dialog)  Indices=[2 3]  OutputSizes=1
  Square1 : Math  Operator=square
  Sum of Elements : Sum  Inputs=+
  Airspeed^2 in yz : Outport
  wires:
  Square1/1 -> Sum of Elements/1
  Selector2/1 -> Square1/1
  Sum of Elements/1 -> Airspeed^2 in yz/1
  Air vector/1 -> Selector2/1

== system Sim1dot0/Subsystem2 ==
  Air vector : Inport
  Selector2 : Selector  InputPortWidth=3  IndexOptions=Index vector (dialog)  Indices=[2 3]  OutputSizes=1
  Square1 : Math  Operator=square
  Sum of Elements : Sum  Inputs=+
  Airspeed^2 in yz : Outport
  wires:
  Square1/1 -> Sum of Elements/1
  Selector2/1 -> Square1/1
  Sum of Elements/1 -> Airspeed^2 in yz/1
  Air vector/1 -> Selector2/1

== system Sim1dot0/Subsystem3 ==
  Air vector : Inport
  Selector2 : Selector  InputPortWidth=3  IndexOptions=Index vector (dialog)  Indices=[2 3]  OutputSizes=1
  Square1 : Math  Operator=square
  Sum of Elements : Sum  Inputs=+
  Airspeed^2 in yz : Outport
  wires:
  Square1/1 -> Sum of Elements/1
  Selector2/1 -> Square1/1
  Sum of Elements/1 -> Airspeed^2 in yz/1
  Air vector/1 -> Selector2/1

== system Sim1dot0/Subsystem4 ==
  Air vector : Inport
  Selector2 : Selector  InputPortWidth=3  IndexOptions=Index vector (dialog)  Indices=[2 3]  OutputSizes=1
  Square1 : Math  Operator=square
  Sum of Elements : Sum  Inputs=+
  Airspeed^2 in yz : Outport
  wires:
  Square1/1 -> Sum of Elements/1
  Selector2/1 -> Square1/1
  Sum of Elements/1 -> Airspeed^2 in yz/1
  Air vector/1 -> Selector2/1

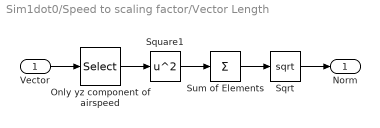
== system Sim1dot0/Speed to scaling factor/Vector Length ==
  Vector : Inport
  Only yz component of airspeed : Selector  InputPortWidth=3  IndexOptions=Index vector (dialog)  Indices=[2 3]  OutputSizes=1
  Sqrt : Sqrt
  Square1 : Math  Operator=square
  Sum of Elements : Sum  Inputs=+
  Norm : Outport
  wires:
  Square1/1 -> Sum of Elements/1
  Sum of Elements/1 -> Sqrt/1
  Vector/1 -> Only yz component of airspeed/1
  Sqrt/1 -> Norm/1
  Only yz component of airspeed/1 -> Square1/1

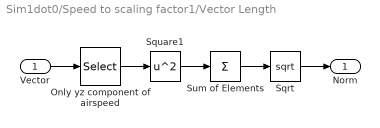
== system Sim1dot0/Speed to scaling factor1/Vector Length ==
  Vector : Inport
  Only yz component of airspeed : Selector  InputPortWidth=3  IndexOptions=Index vector (dialog)  Indices=[2 3]  OutputSizes=1
  Sqrt : Sqrt
  Square1 : Math  Operator=square
  Sum of Elements : Sum  Inputs=+
  Norm : Outport
  wires:
  Square1/1 -> Sum of Elements/1
  Sum of Elements/1 -> Sqrt/1
  Vector/1 -> Only yz component of airspeed/1
  Sqrt/1 -> Norm/1
  Only yz component of airspeed/1 -> Square1/1

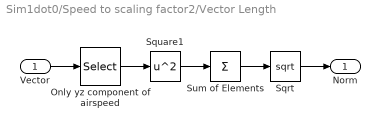
== system Sim1dot0/Speed to scaling factor2/Vector Length ==
  Vector : Inport
  Only yz component of airspeed : Selector  InputPortWidth=3  IndexOptions=Index vector (dialog)  Indices=[2 3]  OutputSizes=1
  Sqrt : Sqrt
  Square1 : Math  Operator=square
  Sum of Elements : Sum  Inputs=+
  Norm : Outport
  wires:
  Square1/1 -> Sum of Elements/1
  Sum of Elements/1 -> Sqrt/1
  Vector/1 -> Only yz component of airspeed/1
  Sqrt/1 -> Norm/1
  Only yz component of airspeed/1 -> Square1/1

== system Sim1dot0/Speed to scaling factor3/Vector Length ==
  Vector : Inport
  Only yz component of airspeed : Selector  InputPortWidth=3  IndexOptions=Index vector (dialog)  Indices=[2 3]  OutputSizes=1
  Sqrt : Sqrt
  Square1 : Math  Operator=square
  Sum of Elements : Sum  Inputs=+
  Norm : Outport
  wires:
  Square1/1 -> Sum of Elements/1
  Sum of Elements/1 -> Sqrt/1
  Vector/1 -> Only yz component of airspeed/1
  Sqrt/1 -> Norm/1
  Only yz component of airspeed/1 -> Square1/1

== matlab function Sim1dot0/F: Fin to body sys ==
  data: fin1 input; vec output; fin2 input; fin3 input; fin4 input
function vec = fcn(fin1, fin2, fin3, fin4)
vx = fin1(1) - fin2(2) - fin3(1) + fin4(2);
vy = fin1(2) + fin2(1) - fin3(2) - fin4(1);
vz = fin1(3) + fin2(3) + fin3(3) + fin4(3);

vec = [vx, vy, vz];

== matlab function Sim1dot0/V air: Body to fin sys ==
  data: v_air_b input; v_f1 output; v_f2 output; v_f3 output; v_f4 output
function [v_f1, v_f2, v_f3, v_f4]= fcn(v_air_b)
vx, vy, vz = v_air_b;
v_f1 = [vx, vy, vz];
v_f2 = [vy, -vx, vz];
v_f3 = [-vx, -vy, vz];
v_f4 = [-vy, vx, vz];

== matlab function Sim1dot0/M: Fin to body sys ==
  data: fin1 input; vec output; fin2 input; fin3 input; fin4 input
function vec = fcn(fin1, fin2, fin3, fin4)
vx = fin1(1) - fin2(2) - fin3(1) + fin4(2);
vy = fin1(2) + fin2(1) - fin3(2) - fin4(1);
vz = fin1(3) + fin2(3) + fin3(3) + fin4(3);

vec = [vx, vy, vz];

== matlab function Sim1dot0/M: Force induced moments on body ==
  data: F1 input; M output; F2 input; F3 input; F4 input
function M = fcn(F1, F2, F3, F4)
r1 = [r_arm_moment, 0, -l_arm_moment];
r2 = [0, r_arm_moment, -l_arm_moment];
r3 = [-r_arm_moment, 0, -l_arm_moment];
r4 = [0, -r_arm_moment, -l_arm_moment];
M = cross(r1, F1) + cross(r2, F2) + cross(r3, F3) + cross(r4, F4);

== matlab function Sim1dot0/Convert fin lift drag to  ==
  data: cl_arr input; F1 output; cd_arr input; F2 output; F3 output; F4 output
function [F1, F2, F3, F4]= fcn(cl_arr, cd_arr)
F1 = [0, cl_arr(1), -cd_arr(1)];
F2 = [0, cl_arr(2), -cd_arr(2)];
F3 = [0, cl_arr(3), -cd_arr(3)];
F4 = [0, cl_arr(4), -cd_arr(4)];

== matlab function Sim1dot0/User sys to Matlab sys ==
  data: M_me input; M_6dof output
function M_6dof = fcn(M_me)
M_6dof = [M_me(3), M_me(1), M_me(2)];

== matlab function Sim1dot0/User sys to Matlab sys1 ==
  data: M_me input; M_6dof output
function M_6dof = fcn(M_me)
M_6dof = [M_me(3), M_me(1), M_me(2)];

== matlab function Sim1dot0/V air: Body to fin sys1 ==
  data: v_air_b input; v_f1 output; v_f2 output; v_f3 output; v_f4 output
function [v_f1, v_f2, v_f3, v_f4]= fcn(v_air_b)
vx, vy, vz = v_air_b;
v_f1 = [vx, vy, vz];
v_f2 = [vy, -vx, vz];
v_f3 = [-vx, -vy, vz];
v_f4 = [-vy, vx, vz];
